simulink model "Target_Control_System"  (R2021b)
settings: Solver=FixedStepDiscrete  StartTime=0.0  StopTime=5  RelTol=1e-3
PreLoadFcn:
  | RTWConfigurationCB('preloadfcn', bdroot);
PostLoadFcn:
  | load('configuration/data_struct.mat');
  | load('configuration/fluxMaps_propMotor.mat');
  | load('configuration/parameterInit_PROP.mat');
  | load('configuration/parameterInit_PUMP.mat');
  | load('configuration/parameterInit_PITCH.mat');
  | load('configuration/parameterInit_TILT.mat');
  | %load('configuration/base_workspace_signal_definition.mat');
  | %load('resolvedatastores_to_baseworkspace_for_faster_simulation.mat');
model workspace (MAT data in the model file):
  SIMULATION_OPTIONS : Simulink.Parameter (value not decoded)
  TARGET_CODE_GEN : Simulink.Parameter (value not decoded)
  TCS_SAMPLE_FREQ_HZ : Simulink.Parameter (value not decoded)
symbols that are objects in the model workspace (value not decoded): TARGET_CODE_GEN, TCS_SAMPLE_FREQ_HZ
undefined symbols (not defined in the file): A_DQ_REF_LPF_INIT__PITCH, A_DQ_REF_LPF_INIT__PROP, A_DQ_REF_LPF_INIT__PUMP, A_DQ_REF_LPF_INIT__TILT, A_OBSERVER_CONFIDENCE_INIT__PITCH, A_OBSERVER_CONFIDENCE_INIT__PROP, A_OBSERVER_CONFIDENCE_INIT__PUMP, A_OBSERVER_CONFIDENCE_INIT__TILT, ACTUATOR_MAX_ANGLE_TRIP__PITCH, ACTUATOR_MIN_ANGLE_TRIP__PITCH, ACTUATOR_POS_SENSOR_INV_DIRECTION__PITCH, ACTUATOR_POS_SENSOR_INV_DIRECTION__TILT, ACTUATOR_POS_SENSOR_OFFSET__PITCH, ACTUATOR_POS_SENSOR_OFFSET__TILT, ADC_scaler1_baseaddr_TILT, ADC_SCALER_FLOAT_TO_FIXPOINT_EXPANSION, ANGLE_ELEC_FROM_SENSOR_OFFSET_INIT__PITCH, ANGLE_ELEC_FROM_SENSOR_OFFSET_INIT__PROP, ANGLE_ELEC_FROM_SENSOR_OFFSET_INIT__PUMP, ANGLE_ELEC_FROM_SENSOR_OFFSET_INIT__TILT, AUTO_CLEAR_FAULTS_ENABLED__PITCH, AUTO_CLEAR_FAULTS_ENABLED__PROP, AUTO_CLEAR_FAULTS_ENABLED__PUMP, AUTO_CLEAR_FAULTS_ENABLED__TILT, AUTO_CLEAR_FAULTS_WAIT_TICKS__PITCH, AUTO_CLEAR_FAULTS_WAIT_TICKS__PROP, AUTO_CLEAR_FAULTS_WAIT_TICKS__PUMP, AUTO_CLEAR_FAULTS_WAIT_TICKS__TILT, AUTO_I_ZERO_IDLE_TICKS__PITCH, AUTO_I_ZERO_IDLE_TICKS__PROP, AUTO_I_ZERO_IDLE_TICKS__PUMP, AUTO_I_ZERO_IDLE_TICKS__TILT, AUTO_I_ZERO_OFFSET_IDC_THRESHOLD__PITCH, AUTO_I_ZERO_OFFSET_IDC_THRESHOLD__PROP, AUTO_I_ZERO_OFFSET_IDC_THRESHOLD__PUMP, AUTO_I_ZERO_OFFSET_IDC_THRESHOLD__TILT, AUTO_I_ZERO_OFFSET_IPH_THRESHOLD__PITCH, AUTO_I_ZERO_OFFSET_IPH_THRESHOLD__PROP, AUTO_I_ZERO_OFFSET_IPH_THRESHOLD__PUMP, AUTO_I_ZERO_OFFSET_IPH_THRESHOLD__TILT, AUTO_SENSORLESS_SWITCHOVER_DISABLE_OMEGA, AUTO_SENSORLESS_SWITCHOVER_ENABLE_OMEGA, AUTO_SENSORLESS_SWITCHOVER_MIN_CONFIDENCE, AUXILIARY_PROTECTION_UNIT_BASEADDR__TILT, blanking_max_error_omega_INIT_PITCH, blanking_max_error_omega_INIT_TILT, blanking_max_error_position_INIT_PITCH, blanking_max_error_position_INIT_TILT, BRUTE_START_I_Q_REF_RAMP_SPEED__PITCH, BRUTE_START_I_Q_REF_RAMP_SPEED__PROP, BRUTE_START_I_Q_REF_RAMP_SPEED__PUMP, BRUTE_START_I_Q_REF_RAMP_SPEED__TILT, CONTROL_LOOP_DT_INIT__PITCH, CONTROL_LOOP_DT_INIT__PROP, CONTROL_LOOP_DT_INIT__PUMP, CONTROL_LOOP_DT_INIT__TILT, CORRECTION_FILTER_SCALE__PITCH, CORRECTION_FILTER_SCALE__PROP, CORRECTION_FILTER_SCALE__PUMP, CORRECTION_FILTER_SCALE__TILT ... (+458)
libraries: simulink x178, Reusables_Lib x24
(part 9 of 47)

== system Target_Control_System/Target_Control_System/Simulation Controls/Simulation Data Store Initialization/setupIirFilters(&oTilt) ==
  setupIirFilters : TriggerPort  TriggerType=function-call  VariantControl=(inherit)  OutputDataType=int8
  Constant : Constant  Value=5000  OutDataTypeStr=single  SampleTime=-1
  Data Store Read : DataStoreRead  DataStoreName=oTilt  DataStoreElements=oTilt.oHw_.fIirDcFInit_  IndexOptions=Index vector (dialog)  Indices=1  OutputSizes=1
  Data Store Read1 : DataStoreRead  DataStoreName=oTilt  DataStoreElements=oTilt.oHw_.fIirFSample_  IndexOptions=Index vector (dialog)  Indices=1  OutputSizes=1
  Data Store Read2 : DataStoreRead  DataStoreName=oTilt  DataStoreElements=oTilt.oHw_.fIirUphaseFInit_  IndexOptions=Index vector (dialog)  Indices=1  OutputSizes=1
  Data Store Read3 : DataStoreRead  DataStoreName=oTilt  DataStoreElements=oTilt.oHw_.fIirIphaseFInit_  IndexOptions=Index vector (dialog)  Indices=1  OutputSizes=1
  Data Store Read5 : DataStoreRead  DataStoreName=oTilt  DataStoreElements=oTilt.oMot_.oState_.fMotorAccelerationStage2Bandwidth_  IndexOptions=Index vector (dialog)  Indices=1  OutputSizes=1
  Data Store Write1 : DataStoreWrite  DataStoreName=oTilt  DataStoreElements=oTilt.oMot_.oParam_.fIdcIirFLpfRads_  IndexOptions=Index vector (dialog)  Indices=1  OutputSizes=1
  Data Store Write11 : DataStoreWrite  DataStoreName=oTilt  DataStoreElements=oTilt.oMot_.oParam_.fUdcIirFLpfRads_  IndexOptions=Index vector (dialog)  Indices=1  OutputSizes=1
  Data Store Write2 : DataStoreWrite  DataStoreName=oTilt  DataStoreElements=oTilt.oMot_.oParam_.fUphaseIirFLpfRads_  IndexOptions=Index vector (dialog)  Indices=1  OutputSizes=1
  Data Store Write3 : DataStoreWrite  DataStoreName=oTilt  DataStoreElements=oTilt.oMot_.oParam_.fIphaseIirFLpfRads_  IndexOptions=Index vector (dialog)  Indices=1  OutputSizes=1
  Data Store Write4 : DataStoreWrite  DataStoreName=oTilt  DataStoreElements=oTilt.oMot_.oState_.fMotorAccelerationStage2Bandwidth_  IndexOptions=Index vector (dialog)  Indices=1  OutputSizes=1
  Gain : Gain  Gain=2*pi
  Gain1 : Gain  Gain=2*pi
  Gain2 : Gain  Gain=2*pi
  computeCoefficientsButter() : Subsystem
  computeCoefficientsButter()1 : Subsystem
  computeCoefficientsButter()2 : Subsystem
  softwareIirFilterInitialize() : Subsystem  Priority=15  TreatAsAtomicUnit=on
  wires:
  Data Store Read/1 -> computeCoefficientsButter()/1(fCutoffFrequencyHz)
  Data Store Read5/1 -> softwareIirFilterInitialize()/1(fFreq3db)
  Gain2/1 -> Data Store Write3/1
  computeCoefficientsButter()2/2(fCutoffFrequencyHz_out) -> Gain2/1
  Data Store Read3/1 -> computeCoefficientsButter()2/1(fCutoffFrequencyHz)
  softwareIirFilterInitialize()/1(fActualFrequencyHz) -> Data Store Write4/1
  computeCoefficientsButter()/2(fCutoffFrequencyHz_out) -> Gain/1
  Data Store Read1/1 -> computeCoefficientsButter()/2(dSampleFrequencyHz), computeCoefficientsButter()1/2(dSampleFrequencyHz), computeCoefficientsButter()2/2(dSampleFrequencyHz)
  Gain1/1 -> Data Store Write2/1
  Gain/1 -> Data Store Write11/1, Data Store Write1/1
  Constant/1 -> softwareIirFilterInitialize()/2(fFreqSample)
  Data Store Read2/1 -> computeCoefficientsButter()1/1(fCutoffFrequencyHz)
  computeCoefficientsButter()1/2(fCutoffFrequencyHz_out) -> Gain1/1

== system Target_Control_System/Target_Control_System/Simulation Controls/Simulation Data Store Initialization/setupIirFilters() ==
  setupIirFilters : TriggerPort  TriggerType=function-call  VariantControl=(inherit)  OutputDataType=int8
  Constant : Constant  Value=5000  OutDataTypeStr=single  SampleTime=-1
  Data Store Read : DataStoreRead  DataStoreName=oPitch  DataStoreElements=oPitch.oHw_.fIirDcFInit_  IndexOptions=Index vector (dialog)  Indices=1  OutputSizes=1
  Data Store Read1 : DataStoreRead  DataStoreName=oPitch  DataStoreElements=oPitch.oHw_.fIirFSample_  IndexOptions=Index vector (dialog)  Indices=1  OutputSizes=1
  Data Store Read2 : DataStoreRead  DataStoreName=oPitch  DataStoreElements=oPitch.oHw_.fIirUphaseFInit_  IndexOptions=Index vector (dialog)  Indices=1  OutputSizes=1
  Data Store Read3 : DataStoreRead  DataStoreName=oPitch  DataStoreElements=oPitch.oHw_.fIirIphaseFInit_  IndexOptions=Index vector (dialog)  Indices=1  OutputSizes=1
  Data Store Read5 : DataStoreRead  DataStoreName=oPitch  DataStoreElements=oPitch.oMot_.oState_.fMotorAccelerationStage2Bandwidth_  IndexOptions=Index vector (dialog)  Indices=1  OutputSizes=1
  Data Store Write1 : DataStoreWrite  DataStoreName=oPitch  DataStoreElements=oPitch.oMot_.oParam_.fIdcIirFLpfRads_  IndexOptions=Index vector (dialog)  Indices=1  OutputSizes=1
  Data Store Write11 : DataStoreWrite  DataStoreName=oPitch  DataStoreElements=oPitch.oMot_.oParam_.fUdcIirFLpfRads_  IndexOptions=Index vector (dialog)  Indices=1  OutputSizes=1
  Data Store Write2 : DataStoreWrite  DataStoreName=oPitch  DataStoreElements=oPitch.oMot_.oParam_.fUphaseIirFLpfRads_  IndexOptions=Index vector (dialog)  Indices=1  OutputSizes=1
  Data Store Write3 : DataStoreWrite  DataStoreName=oPitch  DataStoreElements=oPitch.oMot_.oParam_.fIphaseIirFLpfRads_  IndexOptions=Index vector (dialog)  Indices=1  OutputSizes=1
  Data Store Write4 : DataStoreWrite  DataStoreName=oPitch  DataStoreElements=oPitch.oMot_.oState_.fMotorAccelerationStage2Bandwidth_  IndexOptions=Index vector (dialog)  Indices=1  OutputSizes=1
  Gain : Gain  Gain=2*pi
  Gain1 : Gain  Gain=2*pi
  Gain2 : Gain  Gain=2*pi
  computeCoefficientsButter() : Subsystem
  computeCoefficientsButter()1 : Subsystem
  computeCoefficientsButter()2 : Subsystem
  softwareIirFilterInitialize() : Subsystem  Priority=15  TreatAsAtomicUnit=on
  wires:
  Data Store Read/1 -> computeCoefficientsButter()/1(fCutoffFrequencyHz)
  Data Store Read5/1 -> softwareIirFilterInitialize()/1(fFreq3db)
  Gain2/1 -> Data Store Write3/1
  computeCoefficientsButter()2/2(fCutoffFrequencyHz_out) -> Gain2/1
  Data Store Read3/1 -> computeCoefficientsButter()2/1(fCutoffFrequencyHz)
  softwareIirFilterInitialize()/1(fActualFrequencyHz) -> Data Store Write4/1
  computeCoefficientsButter()/2(fCutoffFrequencyHz_out) -> Gain/1
  Data Store Read1/1 -> computeCoefficientsButter()/2(dSampleFrequencyHz), computeCoefficientsButter()1/2(dSampleFrequencyHz), computeCoefficientsButter()2/2(dSampleFrequencyHz)
  Gain1/1 -> Data Store Write2/1
  Gain/1 -> Data Store Write11/1, Data Store Write1/1
  Constant/1 -> softwareIirFilterInitialize()/2(fFreqSample)
  Data Store Read2/1 -> computeCoefficientsButter()1/1(fCutoffFrequencyHz)
  computeCoefficientsButter()1/2(fCutoffFrequencyHz_out) -> Gain1/1

== system Target_Control_System/Target_Control_System/Simulation Controls/Simulation Data Store Initialization/setupObserver(&oTilt) ==
  setupObserver_Tilt : TriggerPort  TriggerType=function-call  VariantControl=Variant
  Data Store Read : DataStoreRead  DataStoreName=oTilt  DataStoreElements=oTilt.oIsr_.oParam_  IndexOptions=Index vector (dialog)  Indices=1  OutputSizes=1
  Data Store Read1 : DataStoreRead  DataStoreName=oTilt  DataStoreElements=oTilt.oMot_.oParam_  IndexOptions=Index vector (dialog)  Indices=1  OutputSizes=1
  Data Store Write : DataStoreWrite  DataStoreName=oTilt  DataStoreElements=oTilt.oIsr_.oParam_  IndexOptions=Index vector (dialog)  Indices=1  OutputSizes=1
  Data Store Write1 : DataStoreWrite  DataStoreName=oTilt  DataStoreElements=oTilt.oMot_.oParam_  IndexOptions=Index vector (dialog)  Indices=1  OutputSizes=1
  updateObserver_port() : Reusables_Lib/updateObserver_port()  Priority=10  SystemSampleTime=-1  VariantActivationTime=update diagram  Latency=0  AutoFrameSizeCalculation=off
  wires:
  Data Store Read/1 -> updateObserver_port()/1
  Data Store Read1/1 -> updateObserver_port()/2
  updateObserver_port()/1 -> Data Store Write/1
  updateObserver_port()/2 -> Data Store Write1/1

== system Target_Control_System/Target_Control_System/Simulation Controls/Simulation Data Store Initialization/setupObserver() ==
  setupObserver : TriggerPort  TriggerType=function-call  VariantControl=(inherit)  OutputDataType=int8
  Constant : Constant  Value=50000  OutDataTypeStr=single  SampleTime=-1
  Data Store Read : DataStoreRead  DataStoreName=oPitch  DataStoreElements=oPitch.oIsr_.oParam_.fObserverMaxOmegaE_  IndexOptions=Index vector (dialog)  Indices=1  OutputSizes=1
  Data Store Read1 : DataStoreRead  DataStoreName=oPitch  DataStoreElements=oPitch.oIsr_.oParam_.fObserverMaxOmegaEAccel_  IndexOptions=Index vector (dialog)  Indices=1  OutputSizes=1
  Data Store Read2 : DataStoreRead  Priority=5  DataStoreName=oPitch  DataStoreElements=oPitch.oIsr_.oParam_.fControlLoopDt_  IndexOptions=Index vector (dialog)  Indices=1  OutputSizes=1
  Data Store Read3 : DataStoreRead  Priority=5  DataStoreName=oPitch  DataStoreElements=oPitch.oMot_.oParam_.fObserverLoopFilterBandwidthHz_  IndexOptions=Index vector (dialog)  Indices=1  OutputSizes=1
  Data Store Write : DataStoreWrite  DataStoreName=oPitch  DataStoreElements=oPitch.oIsr_.oParam_.oPiDataPll2_.oParameter_.fIntMax_  IndexOptions=Index vector (dialog)  Indices=1  OutputSizes=1
  Data Store Write1 : DataStoreWrite  DataStoreName=oPitch  DataStoreElements=oPitch.oIsr_.oParam_.oPiDataPll2_.oParameter_.fIntMin_  IndexOptions=Index vector (dialog)  Indices=1  OutputSizes=1
  Data Store Write2 : DataStoreWrite  DataStoreName=oPitch  DataStoreElements=oPitch.oIsr_.oParam_.oPiDataPll2_.oParameter_.fOutMin_  IndexOptions=Index vector (dialog)  Indices=1  OutputSizes=1
  Data Store Write3 : DataStoreWrite  DataStoreName=oPitch  DataStoreElements=oPitch.oIsr_.oParam_.oPiDataPll2_.oParameter_.fOutMax_  IndexOptions=Index vector (dialog)  Indices=1  OutputSizes=1
  Data Store Write4 : DataStoreWrite  DataStoreName=oPitch  DataStoreElements=oPitch.oIsr_.oParam_.oPiDataPll2_.oParameter_.fKi_  IndexOptions=Index vector (dialog)  Indices=1  OutputSizes=1
  Gain : Gain  Gain=-1
  Gain1 : Gain  Gain=-1
  updateObserver()_pitch : Subsystem  Priority=10  TreatAsAtomicUnit=on
  wires:
  Gain/1 -> Data Store Write1/1
  Gain1/1 -> Data Store Write2/1
  Data Store Read2/1 -> updateObserver()_pitch/1(oIsr_.oParam_.fControlLoopDt_)
  Data Store Read1/1 -> Gain1/1, Data Store Write3/1
  Constant/1 -> Data Store Write4/1
  Data Store Read/1 -> Gain/1, Data Store Write/1
  Data Store Read3/1 -> updateObserver()_pitch/2(fObserverLoopFilterBandwidthHz_)

== system Target_Control_System/Target_Control_System/Simulation Controls/Simulation Data Store Initialization/setupObserverForPosSensor(&oTilt) ==
  setupObserverForPosSensor : TriggerPort  TriggerType=function-call  VariantControl=(inherit)  OutputDataType=int8
  Data Store Read : DataStoreRead  DataStoreName=oTilt  DataStoreElements=oTilt.oMot_.oParam_.fIntControlLoopDt_  IndexOptions=Index vector (dialog)  Indices=1  OutputSizes=1
  Data Store Read1 : DataStoreRead  DataStoreName=oTilt  DataStoreElements=oTilt.oMot_.oState_.oPosSensor_.fOmegaEDifferentiatorBandwidthHz_  IndexOptions=Index vector (dialog)  Indices=1  OutputSizes=1
  Data Store Write : DataStoreWrite  DataStoreName=oTilt  DataStoreElements=oTilt.oMot_.oState_.oPosSensor_.fOmegaEDifferentiatorBandwidthHz_  IndexOptions=Index vector (dialog)  Indices=1  OutputSizes=1
  softwareIirFilterInitialize() : Subsystem  TreatAsAtomicUnit=on
  wires:
  Data Store Read1/1 -> softwareIirFilterInitialize()/1(fFreq3db)
  softwareIirFilterInitialize()/1(fActualFrequencyHz) -> Data Store Write/1
  Data Store Read/1 -> softwareIirFilterInitialize()/2(fControlLoopDt_)

== system Target_Control_System/Target_Control_System/Simulation Controls/Simulation Data Store Initialization/setupPwm(&oTilt) ==
  setupPwm : TriggerPort  TriggerType=function-call  VariantControl=(inherit)  OutputDataType=int8
  Constant : Constant  Priority=-1  OutDataTypeStr=uint32  SampleTime=-1
  Constant1 : Constant  Priority=-1  Value=0  OutDataTypeStr=uint32  SampleTime=-1
  Data Store Read : DataStoreRead  Priority=-1  DataStoreName=oTilt  DataStoreElements=oTilt.oMot_.oParam_.fPwmFreqKhz_  IndexOptions=Index vector (dialog)  Indices=1  OutputSizes=1
  Data Store Read1 : DataStoreRead  Priority=-1  DataStoreName=oTilt  DataStoreElements=oTilt.oMot_.oState_.fMotorAccelerationStage1Bandwidth_  IndexOptions=Index vector (dialog)  Indices=1  OutputSizes=1
  Data Store Read2 : DataStoreRead  Priority=-1  DataStoreName=oTilt  DataStoreElements=oTilt.oMot_.oState_.fFilterBandwidthForSpeedControlIqRef_  IndexOptions=Index vector (dialog)  Indices=1  OutputSizes=1
  Data Store Write : DataStoreWrite  Priority=-1  DataStoreName=oTilt  DataStoreElements=oTilt.oMot_.oOut_.uiPwmRequestFromMain_  IndexOptions=Index vector (dialog)  Indices=1  OutputSizes=1
  Data Store Write1 : DataStoreWrite  Priority=-1  DataStoreName=oTilt  DataStoreElements=oTilt.oMot_.oOut_.uiPwmDutyTicksFromMainA_  IndexOptions=Index vector (dialog)  Indices=1  OutputSizes=1
  Data Store Write2 : DataStoreWrite  Priority=-1  DataStoreName=oTilt  DataStoreElements=oTilt.oMot_.oOut_.uiPwmDutyTicksFromMainB_  IndexOptions=Index vector (dialog)  Indices=1  OutputSizes=1
  Data Store Write4 : DataStoreWrite  Priority=-1  DataStoreName=oTilt  DataStoreElements=oTilt.oMot_.oOut_.uiPwmDutyTicksFromMainC_  IndexOptions=Index vector (dialog)  Indices=1  OutputSizes=1
  setPwmFrequencyApplication()_tilt : Subsystem  Priority=1  TreatAsAtomicUnit=on
  wires:
  Data Store Read/1 -> setPwmFrequencyApplication()_tilt/1(fPwmFreqKhz_)
  Data Store Read1/1 -> setPwmFrequencyApplication()_tilt/2(fMotorAccelerationStage1Bandwidth_)
  Data Store Read2/1 -> setPwmFrequencyApplication()_tilt/3(fFilterBandwidthForSpeedControlIqRef_)
  Constant1/1 -> Data Store Write1/1, Data Store Write2/1, Data Store Write4/1
  Constant/1 -> Data Store Write/1

== system Target_Control_System/Target_Control_System/Simulation Controls/Simulation Data Store Initialization/setupPwm() ==
  setupPwm : TriggerPort  TriggerType=function-call  VariantControl=(inherit)  OutputDataType=int8
  Constant : Constant  Priority=-1  OutDataTypeStr=uint32  SampleTime=-1
  Constant1 : Constant  Priority=-1  Value=0  OutDataTypeStr=uint32  SampleTime=-1
  Data Store Read : DataStoreRead  Priority=-1  DataStoreName=oPitch  DataStoreElements=oPitch.oMot_.oParam_.fPwmFreqKhz_  IndexOptions=Index vector (dialog)  Indices=1  OutputSizes=1
  Data Store Read1 : DataStoreRead  Priority=-1  DataStoreName=oPitch  DataStoreElements=oPitch.oMot_.oState_.fMotorAccelerationStage1Bandwidth_  IndexOptions=Index vector (dialog)  Indices=1  OutputSizes=1
  Data Store Read2 : DataStoreRead  Priority=-1  DataStoreName=oPitch  DataStoreElements=oPitch.oMot_.oState_.fFilterBandwidthForSpeedControlIqRef_  IndexOptions=Index vector (dialog)  Indices=1  OutputSizes=1
  Data Store Write : DataStoreWrite  Priority=-1  DataStoreName=oPitch  DataStoreElements=oPitch.oMot_.oOut_.uiPwmRequestFromMain_  IndexOptions=Index vector (dialog)  Indices=1  OutputSizes=1
  Data Store Write1 : DataStoreWrite  Priority=-1  DataStoreName=oPitch  DataStoreElements=oPitch.oMot_.oOut_.uiPwmDutyTicksFromMainA_  IndexOptions=Index vector (dialog)  Indices=1  OutputSizes=1
  Data Store Write2 : DataStoreWrite  Priority=-1  DataStoreName=oPitch  DataStoreElements=oPitch.oMot_.oOut_.uiPwmDutyTicksFromMainB_  IndexOptions=Index vector (dialog)  Indices=1  OutputSizes=1
  Data Store Write4 : DataStoreWrite  Priority=-1  DataStoreName=oPitch  DataStoreElements=oPitch.oMot_.oOut_.uiPwmDutyTicksFromMainC_  IndexOptions=Index vector (dialog)  Indices=1  OutputSizes=1
  setPwmFrequencyApplication()_pitch : Subsystem  Priority=1  TreatAsAtomicUnit=on
  wires:
  Data Store Read/1 -> setPwmFrequencyApplication()_pitch/1(fPwmFreqKhz_)
  Data Store Read1/1 -> setPwmFrequencyApplication()_pitch/2(fMotorAccelerationStage1Bandwidth_)
  Data Store Read2/1 -> setPwmFrequencyApplication()_pitch/3(fFilterBandwidthForSpeedControlIqRef_)
  Constant1/1 -> Data Store Write1/1, Data Store Write2/1, Data Store Write4/1
  Constant/1 -> Data Store Write/1

== system Target_Control_System/Target_Control_System/Simulation Controls/Simulation Data Store Initialization/updateIqSetpointMax(&oTilt) ==
  updateIqSetpointMax : TriggerPort  TriggerType=function-call  VariantControl=(inherit)  OutputDataType=int8
  Add : Sum
  Constant : Constant  OutDataTypeStr=single  SampleTime=-1
  Constant1 : Constant  Value=0  OutDataTypeStr=single  SampleTime=-1
  Constant2 : Constant  Value=0  OutDataTypeStr=single  SampleTime=-1
  Data Store Read : DataStoreRead  DataStoreName=oTilt  DataStoreElements=oTilt.oMot_.oParam_.fISetpointMax_  IndexOptions=Index vector (dialog)  Indices=1  OutputSizes=1
  Data Store Read1 : DataStoreRead  DataStoreName=oTilt  DataStoreElements=oTilt.oMot_.oParam_.fIdRefFractionOfIq_  IndexOptions=Index vector (dialog)  Indices=1  OutputSizes=1
  Data Store Read2 : DataStoreRead  DataStoreName=oTilt  DataStoreElements=oTilt.oMot_.oParam_.fTorqueAuthorityFraction_  IndexOptions=Index vector (dialog)  Indices=1  OutputSizes=1
  Data Store Read3 : DataStoreRead  DataStoreName=oTilt  DataStoreElements=oTilt.oMot_.oParam_.oPiDataRpm_.oParameter_.fIntMin_  IndexOptions=Index vector (dialog)  Indices=1  OutputSizes=1
  Data Store Read4 : DataStoreRead  DataStoreName=oTilt  DataStoreElements=oTilt.oMot_.oParam_.oPiDataRpm_.oParameter_.fOutMin_  IndexOptions=Index vector (dialog)  Indices=1  OutputSizes=1
  Data Store Write : DataStoreWrite  DataStoreName=oTilt  DataStoreElements=oTilt.oMot_.oParam_.fIqSetpointMax_  IndexOptions=Index vector (dialog)  Indices=1  OutputSizes=1
  Data Store Write1 : DataStoreWrite  DataStoreName=oTilt  DataStoreElements=oTilt.oMot_.oParam_.oPiDataRpm_.oParameter_.fIntMax_  IndexOptions=Index vector (dialog)  Indices=1  OutputSizes=1
  Data Store Write10 : DataStoreWrite  DataStoreName=oTilt  DataStoreElements=oTilt.oMot_.oParam_.oPid2DataRpmCtrl_.oParameter_.fDMax_  IndexOptions=Index vector (dialog)  Indices=1  OutputSizes=1
  Data Store Write2 : DataStoreWrite  DataStoreName=oTilt  DataStoreElements=oTilt.oMot_.oParam_.oPiDataRpm_.oParameter_.fIntMin_  IndexOptions=Index vector (dialog)  Indices=1  OutputSizes=1
  Data Store Write3 : DataStoreWrite  DataStoreName=oTilt  DataStoreElements=oTilt.oMot_.oParam_.oPiDataRpm_.oParameter_.fOutMax_  IndexOptions=Index vector (dialog)  Indices=1  OutputSizes=1
  Data Store Write4 : DataStoreWrite  DataStoreName=oTilt  DataStoreElements=oTilt.oMot_.oParam_.oPiDataRpm_.oParameter_.fOutMin_  IndexOptions=Index vector (dialog)  Indices=1  OutputSizes=1
  Data Store Write5 : DataStoreWrite  DataStoreName=oTilt  DataStoreElements=oTilt.oMot_.oParam_.oPid2DataRpmCtrl_.oParameter_.fIntMin_  IndexOptions=Index vector (dialog)  Indices=1  OutputSizes=1
  Data Store Write6 : DataStoreWrite  DataStoreName=oTilt  DataStoreElements=oTilt.oMot_.oParam_.oPid2DataRpmCtrl_.oParameter_.fIntMax_  IndexOptions=Index vector (dialog)  Indices=1  OutputSizes=1
  Data Store Write7 : DataStoreWrite  DataStoreName=oTilt  DataStoreElements=oTilt.oMot_.oParam_.oPid2DataRpmCtrl_.oParameter_.fOutMin_  IndexOptions=Index vector (dialog)  Indices=1  OutputSizes=1
  Data Store Write8 : DataStoreWrite  DataStoreName=oTilt  DataStoreElements=oTilt.oMot_.oParam_.oPid2DataRpmCtrl_.oParameter_.fOutMax_  IndexOptions=Index vector (dialog)  Indices=1  OutputSizes=1
  Data Store Write9 : DataStoreWrite  DataStoreName=oTilt  DataStoreElements=oTilt.oMot_.oParam_.oPid2DataRpmCtrl_.oParameter_.fDMin_  IndexOptions=Index vector (dialog)  Indices=1  OutputSizes=1
  Divide : Product  Inputs=**
  Divide1 : Product  Inputs=**/
  Gain{,1..4} (5 alike) : Gain  Gain=-1
  Relational Operator : RelationalOperator  Operator===  OutDataTypeStr=boolean  RndMeth=Simplest
  Relational Operator1 : RelationalOperator  Operator===  OutDataTypeStr=boolean  RndMeth=Simplest
  Sqrt : Sqrt  SaturateOnIntegerOverflow=on
  Switch : Switch  Criteria=u2 > Threshold
  Switch1 : Switch  Criteria=u2 > Threshold
  wires:
  Sqrt/1 -> Divide1/3
  Data Store Read3/1 -> Relational Operator/1, Switch/1
  Data Store Read1/1 -> Divide/1, Divide/2
  Data Store Read/1 -> Divide1/2
  Constant1/1 -> Relational Operator/2
  Add/1 -> Sqrt/1
  Constant/1 -> Add/2
  Relational Operator1/1 -> Switch1/2
  Gain/1 -> Switch/3
  Divide1/1 -> Data Store Write3/1, Data Store Write6/1, Data Store Write8/1, Data Store Write10/1, Gain4/1, Gain3/1, Gain2/1, Data Store Write1/1, Data Store Write/1, Gain/1, Gain1/1
  Relational Operator/1 -> Switch/2
  Divide/1 -> Add/1
  Switch1/1 -> Data Store Write4/1
  Switch/1 -> Data Store Write2/1
  Constant2/1 -> Relational Operator1/2
  Data Store Read4/1 -> Relational Operator1/1, Switch1/1
  Gain4/1 -> Data Store Write9/1
  Gain1/1 -> Switch1/3
  Gain3/1 -> Data Store Write7/1
  Data Store Read2/1 -> Divide1/1
  Gain2/1 -> Data Store Write5/1

== system Target_Control_System/Target_Control_System/Simulation Controls/Simulation Data Store Initialization/updateIqSetpointMax() ==
  updateIqSetpointMax : TriggerPort  TriggerType=function-call  VariantControl=(inherit)  OutputDataType=int8
  Add : Sum
  Constant : Constant  OutDataTypeStr=single  SampleTime=-1
  Constant1 : Constant  Value=0  OutDataTypeStr=single  SampleTime=-1
  Constant2 : Constant  Value=0  OutDataTypeStr=single  SampleTime=-1
  Data Store Read : DataStoreRead  DataStoreName=oPitch  DataStoreElements=oPitch.oMot_.oParam_.fISetpointMax_  IndexOptions=Index vector (dialog)  Indices=1  OutputSizes=1
  Data Store Read1 : DataStoreRead  DataStoreName=oPitch  DataStoreElements=oPitch.oMot_.oParam_.fIdRefFractionOfIq_  IndexOptions=Index vector (dialog)  Indices=1  OutputSizes=1
  Data Store Read2 : DataStoreRead  DataStoreName=oPitch  DataStoreElements=oPitch.oMot_.oParam_.fTorqueAuthorityFraction_  IndexOptions=Index vector (dialog)  Indices=1  OutputSizes=1
  Data Store Read3 : DataStoreRead  DataStoreName=oPitch  DataStoreElements=oPitch.oMot_.oParam_.oPiDataRpm_.oParameter_.fIntMin_  IndexOptions=Index vector (dialog)  Indices=1  OutputSizes=1
  Data Store Read4 : DataStoreRead  DataStoreName=oPitch  DataStoreElements=oPitch.oMot_.oParam_.oPiDataRpm_.oParameter_.fOutMin_  IndexOptions=Index vector (dialog)  Indices=1  OutputSizes=1
  Data Store Write : DataStoreWrite  DataStoreName=oPitch  DataStoreElements=oPitch.oMot_.oParam_.fIqSetpointMax_  IndexOptions=Index vector (dialog)  Indices=1  OutputSizes=1
  Data Store Write1 : DataStoreWrite  DataStoreName=oPitch  DataStoreElements=oPitch.oMot_.oParam_.oPiDataRpm_.oParameter_.fIntMax_  IndexOptions=Index vector (dialog)  Indices=1  OutputSizes=1
  Data Store Write10 : DataStoreWrite  DataStoreName=oPitch  DataStoreElements=oPitch.oMot_.oParam_.oPid2DataRpmCtrl_.oParameter_.fDMax_  IndexOptions=Index vector (dialog)  Indices=1  OutputSizes=1
  Data Store Write2 : DataStoreWrite  DataStoreName=oPitch  DataStoreElements=oPitch.oMot_.oParam_.oPiDataRpm_.oParameter_.fIntMin_  IndexOptions=Index vector (dialog)  Indices=1  OutputSizes=1
  Data Store Write3 : DataStoreWrite  DataStoreName=oPitch  DataStoreElements=oPitch.oMot_.oParam_.oPiDataRpm_.oParameter_.fOutMax_  IndexOptions=Index vector (dialog)  Indices=1  OutputSizes=1
  Data Store Write4 : DataStoreWrite  DataStoreName=oPitch  DataStoreElements=oPitch.oMot_.oParam_.oPiDataRpm_.oParameter_.fOutMin_  IndexOptions=Index vector (dialog)  Indices=1  OutputSizes=1
  Data Store Write5 : DataStoreWrite  DataStoreName=oPitch  DataStoreElements=oPitch.oMot_.oParam_.oPid2DataRpmCtrl_.oParameter_.fIntMin_  IndexOptions=Index vector (dialog)  Indices=1  OutputSizes=1
  Data Store Write6 : DataStoreWrite  DataStoreName=oPitch  DataStoreElements=oPitch.oMot_.oParam_.oPid2DataRpmCtrl_.oParameter_.fIntMax_  IndexOptions=Index vector (dialog)  Indices=1  OutputSizes=1
  Data Store Write7 : DataStoreWrite  DataStoreName=oPitch  DataStoreElements=oPitch.oMot_.oParam_.oPid2DataRpmCtrl_.oParameter_.fOutMin_  IndexOptions=Index vector (dialog)  Indices=1  OutputSizes=1
  Data Store Write8 : DataStoreWrite  DataStoreName=oPitch  DataStoreElements=oPitch.oMot_.oParam_.oPid2DataRpmCtrl_.oParameter_.fOutMax_  IndexOptions=Index vector (dialog)  Indices=1  OutputSizes=1
  Data Store Write9 : DataStoreWrite  DataStoreName=oPitch  DataStoreElements=oPitch.oMot_.oParam_.oPid2DataRpmCtrl_.oParameter_.fDMin_  IndexOptions=Index vector (dialog)  Indices=1  OutputSizes=1
  Divide : Product  Inputs=**
  Divide1 : Product  Inputs=**/
  Gain{,1..4} (5 alike) : Gain  Gain=-1
  Relational Operator : RelationalOperator  Operator===  OutDataTypeStr=boolean  RndMeth=Simplest
  Relational Operator1 : RelationalOperator  Operator===  OutDataTypeStr=boolean  RndMeth=Simplest
  Sqrt : Sqrt  SaturateOnIntegerOverflow=on
  Switch : Switch  Criteria=u2 > Threshold
  Switch1 : Switch  Criteria=u2 > Threshold
  wires:
  Sqrt/1 -> Divide1/3
  Data Store Read3/1 -> Relational Operator/1, Switch/1
  Data Store Read1/1 -> Divide/1, Divide/2
  Data Store Read/1 -> Divide1/2
  Constant1/1 -> Relational Operator/2
  Add/1 -> Sqrt/1
  Constant/1 -> Add/2
  Relational Operator1/1 -> Switch1/2
  Gain/1 -> Switch/3
  Divide1/1 -> Data Store Write3/1, Data Store Write6/1, Data Store Write8/1, Data Store Write10/1, Gain4/1, Gain3/1, Gain2/1, Data Store Write1/1, Data Store Write/1, Gain/1, Gain1/1
  Relational Operator/1 -> Switch/2
  Divide/1 -> Add/1
  Switch1/1 -> Data Store Write4/1
  Switch/1 -> Data Store Write2/1
  Constant2/1 -> Relational Operator1/2
  Data Store Read4/1 -> Relational Operator1/1, Switch1/1
  Gain4/1 -> Data Store Write9/1
  Gain1/1 -> Switch1/3
  Gain3/1 -> Data Store Write7/1
  Data Store Read2/1 -> Divide1/1
  Gain2/1 -> Data Store Write5/1

== system Target_Control_System/Target_Control_System/Simulation Controls/Simulation Data Store Initialization/updateServoObserver(&oTilt) ==
  updateServoObserver : TriggerPort  TriggerType=function-call  VariantControl=(inherit)  OutputDataType=int8
  Data Store Read : DataStoreRead  DataStoreName=oTilt  DataStoreElements=oTilt.oMot_.oParam_.fIntControlLoopDt_  IndexOptions=Index vector (dialog)  Indices=1  OutputSizes=1
  Data Store Read1 : DataStoreRead  DataStoreName=oTilt  DataStoreElements=oTilt.oMot_.oState_.oPosSensor_.fOmegaEDifferentiatorBandwidthHz_  IndexOptions=Index vector (dialog)  Indices=1  OutputSizes=1
  updateServoObserver() : Subsystem  Priority=10  TreatAsAtomicUnit=on
  wires:
  Data Store Read1/1 -> updateServoObserver()/2(fOmegaEDifferentiatorBandwidthHz_)
  Data Store Read/1 -> updateServoObserver()/1(oIsr_.oParam_.fControlLoopDt_)

== system Target_Control_System/Target_Control_System/Simulation Controls/Simulation Data Store Initialization/updateServoObserver() ==
  updateServoObserver : TriggerPort  TriggerType=function-call  VariantControl=(inherit)  OutputDataType=int8
  Data Store Read : DataStoreRead  DataStoreName=oPitch  DataStoreElements=oPitch.oMot_.oParam_.fIntControlLoopDt_  IndexOptions=Index vector (dialog)  Indices=1  OutputSizes=1
  Data Store Read1 : DataStoreRead  DataStoreName=oPitch  DataStoreElements=oPitch.oMot_.oState_.oPosSensor_.fOmegaEDifferentiatorBandwidthHz_  IndexOptions=Index vector (dialog)  Indices=1  OutputSizes=1
  updateServoObserver()_pitch : Subsystem  Priority=10  TreatAsAtomicUnit=on
  wires:
  Data Store Read1/1 -> updateServoObserver()_pitch/2(fOmegaEDifferentiatorBandwidthHz_)
  Data Store Read/1 -> updateServoObserver()_pitch/1(oIsr_.oParam_.fControlLoopDt_)

== system Target_Control_System/Target_Control_System/Simulation Controls/Simulation Data Store Initialization/updateSoftCurrentLimitTilt()1 ==
  updateSoftCurrentLimitTilt : TriggerPort  TriggerType=function-call  VariantControl=Variant

== system Target_Control_System/Target_Control_System/Simulation Controls/pitchMotor/Apply Simulation Parameter Values ==
  OneOverSensorPolePairs : Inport
  Data Store Write : DataStoreWrite  DataStoreName=oPitch  DataStoreElements=oPitch.oMot_.oParam_.fOneOverSensorPolepairs_  IndexOptions=Index vector (dialog)  Indices=1  OutputSizes=1
  wires:
  OneOverSensorPolePairs/1 -> Data Store Write/1

== system Target_Control_System/Target_Control_System/Simulation Controls/pitchMotor/Apply Simulation Setpoints ==
  controllerSelection : Inport
  Current Setpoint for Simulation : Inport  Port=2
  Speed Setpoint for Simulation : Inport  Port=3
  Position Setpoint for Simulation : Inport  Port=4
  Constant : Constant  OutDataTypeStr=uint32  SampleTime=-1
  Constant1 : Constant  Value=3  OutDataTypeStr=uint32  SampleTime=-1
  Constant3 : Constant  Value=2  OutDataTypeStr=uint32  SampleTime=-1
  Equal : RelationalOperator  Operator===  OutDataTypeStr=boolean  RndMeth=Simplest
  Equal1 : RelationalOperator  Operator===  OutDataTypeStr=boolean  RndMeth=Simplest
  Equal2 : RelationalOperator  Operator===  OutDataTypeStr=boolean  RndMeth=Simplest
  Set Current : Subsystem  TreatAsAtomicUnit=on
  Set Position : Subsystem  TreatAsAtomicUnit=on
  Set Speed : Subsystem  TreatAsAtomicUnit=on
  wires:
  Position Setpoint for Simulation/1 -> Set Position/1(Position Setpoint for Simulation)
  Speed Setpoint for Simulation/1 -> Set Speed/1(Speed Setpoint for Simulation)
  Current Setpoint for Simulation/1 -> Set Current/1(Current Setpoint for Simulation)
  Equal2/1 -> Set Position/Enable
  Constant1/1 -> Equal2/2
  controllerSelection/1 -> Equal/1, Equal1/1, Equal2/1
  Equal1/1 -> Set Speed/Enable
  Constant3/1 -> Equal1/2
  Constant/1 -> Equal/2
  Equal/1 -> Set Current/Enable

== system Target_Control_System/Target_Control_System/Simulation Controls/pitchMotor/Drive Enable ==
  pitchMotor_uiEnable : Inport
  Trigger : TriggerPort  TriggerType=falling  VariantControl=Variant
  Data Store Write43 : DataStoreWrite  DataStoreName=oPitch  DataStoreElements=oPitch.oMot_.oOut_.uiEnable_  IndexOptions=Index vector (dialog)  Indices=1  OutputSizes=1
  wires:
  pitchMotor_uiEnable/1 -> Data Store Write43/1

== system Target_Control_System/Target_Control_System/Simulation Controls/pitchMotor/Initialize controller ==
  controllerSelection : Inport
  Trigger : TriggerPort  TriggerType=falling  VariantControl=Variant  PortDimensions=1
  Constant : Constant  OutDataTypeStr=uint32  SampleTime=-1
  Constant1 : Constant  Value=3  OutDataTypeStr=uint32  SampleTime=-1
  Constant3 : Constant  Value=2  OutDataTypeStr=uint32  SampleTime=-1
  Equal : RelationalOperator  Operator===  OutDataTypeStr=boolean  RndMeth=Simplest
  Equal1 : RelationalOperator  Operator===  OutDataTypeStr=boolean  RndMeth=Simplest
  Equal2 : RelationalOperator  Operator===  OutDataTypeStr=boolean  RndMeth=Simplest
  Set Current Controller : Subsystem  TreatAsAtomicUnit=on
  Set Position Controller : Subsystem  TreatAsAtomicUnit=on
  Set Speed Controller : Subsystem  TreatAsAtomicUnit=on
  wires:
  Equal2/1 -> Set Position Controller/Enable
  Constant1/1 -> Equal2/2
  controllerSelection/1 -> Equal/1, Equal1/1, Equal2/1
  Equal1/1 -> Set Speed Controller/Enable
  Constant3/1 -> Equal1/2
  Constant/1 -> Equal/2
  Equal/1 -> Set Current Controller/Enable

== system Target_Control_System/Target_Control_System/Simulation Controls/propMotor/Drive Enable ==
  propMotor_uiEnable : Inport
  Trigger : TriggerPort  TriggerType=falling  VariantControl=Variant
  Data Store Write43 : DataStoreWrite  DataStoreName=oProp  DataStoreElements=oProp.oMot_.oOut_.uiEnable_  IndexOptions=Index vector (dialog)  Indices=1  OutputSizes=1
  wires:
  propMotor_uiEnable/1 -> Data Store Write43/1

== system Target_Control_System/Target_Control_System/Simulation Controls/pumpMotor/Drive Enable ==
  pumpMotor_uiEnable : Inport
  Trigger : TriggerPort  TriggerType=falling  VariantControl=Variant
  Data Store Write43 : DataStoreWrite  DataStoreName=oPump  DataStoreElements=oPump.oMot_.oOut_.uiEnable_  IndexOptions=Index vector (dialog)  Indices=1  OutputSizes=1
  wires:
  pumpMotor_uiEnable/1 -> Data Store Write43/1

== system Target_Control_System/Target_Control_System/Simulation Controls/tiltMotor/Apply Simulation Parameter Values ==
  OneOverSensorPolePairs : Inport
  TiltReadheadCompensationEnabled : Inport  Port=2
  Data Store Write : DataStoreWrite  DataStoreName=oTilt  DataStoreElements=oTilt.oMot_.oParam_.fOneOverSensorPolepairs_  IndexOptions=Index vector (dialog)  Indices=1  OutputSizes=1
  Data Store Write1 : DataStoreWrite  DataStoreName=oTilt  DataStoreElements=oTilt.oMot_.oState_.oPosSensor_.iTiltReadheadCompensationEnabled_  IndexOptions=Index vector (dialog)  Indices=1  OutputSizes=1
  wires:
  TiltReadheadCompensationEnabled/1 -> Data Store Write1/1
  OneOverSensorPolePairs/1 -> Data Store Write/1

== system Target_Control_System/Target_Control_System/Simulation Controls/tiltMotor/Apply Simulation Setpoints ==
  controllerSelection : Inport
  Current Setpoint for Simulation : Inport  Port=2
  Speed Setpoint for Simulation : Inport  Port=3
  Position Setpoint for Simulation : Inport  Port=4
  Constant : Constant  OutDataTypeStr=uint32  SampleTime=-1
  Constant1 : Constant  Value=3  OutDataTypeStr=uint32  SampleTime=-1
  Constant3 : Constant  Value=2  OutDataTypeStr=uint32  SampleTime=-1
  Equal : RelationalOperator  Operator===  OutDataTypeStr=boolean  RndMeth=Simplest
  Equal1 : RelationalOperator  Operator===  OutDataTypeStr=boolean  RndMeth=Simplest
  Equal2 : RelationalOperator  Operator===  OutDataTypeStr=boolean  RndMeth=Simplest
  Set Current : Subsystem  TreatAsAtomicUnit=on
  Set Position : Subsystem  TreatAsAtomicUnit=on
  Set Speed : Subsystem  TreatAsAtomicUnit=on
  wires:
  Position Setpoint for Simulation/1 -> Set Position/1(Position Setpoint for Simulation)
  Speed Setpoint for Simulation/1 -> Set Speed/1(Speed Setpoint for Simulation)
  Current Setpoint for Simulation/1 -> Set Current/1(Current Setpoint for Simulation)
  Equal2/1 -> Set Position/Enable
  Constant1/1 -> Equal2/2
  controllerSelection/1 -> Equal/1, Equal1/1, Equal2/1
  Equal1/1 -> Set Speed/Enable
  Constant3/1 -> Equal1/2
  Constant/1 -> Equal/2
  Equal/1 -> Set Current/Enable

== system Target_Control_System/Target_Control_System/Simulation Controls/tiltMotor/Drive Enable ==
  tiltMotor_uiEnable : Inport
  Trigger : TriggerPort  TriggerType=falling  VariantControl=Variant
  Data Store Write43 : DataStoreWrite  DataStoreName=oTilt  DataStoreElements=oTilt.oMot_.oOut_.uiEnable_  IndexOptions=Index vector (dialog)  Indices=1  OutputSizes=1
  wires:
  tiltMotor_uiEnable/1 -> Data Store Write43/1

== system Target_Control_System/Target_Control_System/Simulation Controls/tiltMotor/Initialize controller ==
  controllerSelection : Inport
  Trigger : TriggerPort  TriggerType=falling  VariantControl=Variant  PortDimensions=1
  Constant : Constant  OutDataTypeStr=uint32  SampleTime=-1
  Constant1 : Constant  Value=3  OutDataTypeStr=uint32  SampleTime=-1
  Constant3 : Constant  Value=2  OutDataTypeStr=uint32  SampleTime=-1
  Equal : RelationalOperator  Operator===  OutDataTypeStr=boolean  RndMeth=Simplest
  Equal1 : RelationalOperator  Operator===  OutDataTypeStr=boolean  RndMeth=Simplest
  Equal2 : RelationalOperator  Operator===  OutDataTypeStr=boolean  RndMeth=Simplest
  Set Current Controller : Subsystem  TreatAsAtomicUnit=on
  Set Position Controller : Subsystem  TreatAsAtomicUnit=on
  Set Speed Controller : Subsystem  TreatAsAtomicUnit=on
  wires:
  Constant3/1 -> Equal1/2
  Equal2/1 -> Set Position Controller/Enable
  Equal/1 -> Set Current Controller/Enable
  Constant1/1 -> Equal2/2
  Constant/1 -> Equal/2
  Equal1/1 -> Set Speed Controller/Enable
  controllerSelection/1 -> Equal/1, Equal1/1, Equal2/1

== system Target_Control_System/Target_Control_System/InterruptFunction/pitchMotor_dataToMain/Variant Subsystem/Subsystem1 ==

== system Target_Control_System/Target_Control_System/InterruptFunction/pitchMotor_dataToMain/Variant Subsystem/VP_leader_follower_postion_copy ==
  Constant3 : Constant  Value=true
  Data Store Read24 : DataStoreRead  DataStoreName=oPitch  DataStoreElements=oPitch.oMot_.oParam_.uiSlaveRole_  IndexOptions=Index vector (dialog)  Indices=1  OutputSizes=1
  Follower Postion Enabled Subsystem : Subsystem  TreatAsAtomicUnit=on
  Leader Postion Enabled Subsystem : Subsystem  TreatAsAtomicUnit=on
  NOT1 : Logic  Operator=NOT  IconShape=distinctive  AllPortsSameDT=off  OutDataTypeStr=boolean
  Relational Operator : RelationalOperator  Operator===  OutDataTypeStr=boolean  RndMeth=Simplest
  wires:
  NOT1/1 -> Follower Postion Enabled Subsystem/Enable
  Relational Operator/1 -> Leader Postion Enabled Subsystem/Enable, NOT1/1
  Data Store Read24/1 -> Relational Operator/1
  Constant3/1 -> Relational Operator/2

== system Target_Control_System/Target_Control_System/InterruptFunction/pitchMotor_isrTask/abcToAlphaBeta/Alpha-Beta Calcs1 ==
  iInverseDirection : Inport
  fIa : Inport  Port=2
  fIb : Inport  Port=3
  fIc : Inport  Port=4
  fUaPostlpf : Inport  Port=5
  fUbPostlpf : Inport  Port=6
  fUcPostlpf : Inport  Port=7
  Demux1 : Demux  Outputs=2
  Demux4 : Demux  Outputs=2
  Mux1 : Mux  Inputs=3
  Mux3 : Mux  Inputs=3
  Switch : Switch  Criteria=u2 > Threshold
  Switch1 : Switch  Criteria=u2 > Threshold
  abc to alpha/beta1 : Gain  Gain="2/3*[1 -0.5 -0.5  ; 0 sqrt(3)/2 -sqrt(3)/2 ]"  Multiplication=Matrix(K*u) (u vector)
  abc to alpha/beta4 : Gain  Gain="2/3*[1 -0.5 -0.5  ; 0 sqrt(3)/2 -sqrt(3)/2 ]"  Multiplication=Matrix(K*u) (u vector)
  abc to alpha/beta_inverseDirection : Gain  Gain="2/3*[1 -0.5 -0.5  ; 0 -sqrt(3)/2 sqrt(3)/2 ]"  Multiplication=Matrix(K*u) (u vector)
  abc to alpha/beta_inverseDirection1 : Gain  Gain="2/3*[1 -0.5 -0.5  ; 0 -sqrt(3)/2 sqrt(3)/2 ]"  Multiplication=Matrix(K*u) (u vector)
  fIAlpha : Outport
  fIBeta : Outport  Port=2
  fUAlpha : Outport  Port=3
  fUBeta : Outport  Port=4
  wires:
  Demux4/1 -> fIAlpha/1
  Demux1/1 -> fUAlpha/1
  Demux1/2 -> fUBeta/1
  fIa/1 -> Mux1/1
  abc to alpha/beta1/1 -> Switch1/3
  abc to alpha/beta_inverseDirection1/1 -> Switch1/1
  Demux4/2 -> fIBeta/1
  Mux3/1 -> abc to alpha/beta_inverseDirection1/1, abc to alpha/beta1/1
  fUcPostlpf/1 -> Mux3/3
  fUbPostlpf/1 -> Mux3/2
  abc to alpha/beta_inverseDirection/1 -> Switch/1
  Switch1/1 -> Demux1/1
  abc to alpha/beta4/1 -> Switch/3
  fIc/1 -> Mux1/3
  Switch/1 -> Demux4/1
  iInverseDirection/1 -> Switch1/2, Switch/2
  Mux1/1 -> abc to alpha/beta4/1, abc to alpha/beta_inverseDirection/1
  fIb/1 -> Mux1/2
  fUaPostlpf/1 -> Mux3/1

== system Target_Control_System/Target_Control_System/InterruptFunction/pitchMotor_isrTask/abcToAlphaBeta/Calc Angle From Speed ==
  Omega : Inport
  Integrator with Angle Wrapper : Subsystem
  Integrator with Angle Wrapper_OLD : Subsystem  Commented=on
  fFluxMainAngleRaw2 : Outport
  wires:
  Omega/1 -> Integrator with Angle Wrapper/1(Omega)
  Integrator with Angle Wrapper/1(Angle) -> fFluxMainAngleRaw2/1  "fFluxMainAngleRaw2_"

== system Target_Control_System/Target_Control_System/InterruptFunction/pitchMotor_isrTask/abcToAlphaBeta/ModelSource ==
  note: 1) Add Subsystem or Model blocks as valid variant choices.
      | 2) You cannot connect blocks at this level. At simulation, connectivity is automatically
      | determined, based on the active variant and port name matching.
  DoNotIncludeCustomCode : Subsystem  TreatAsAtomicUnit=on  VariantControl=TARGET_CODE_GEN == 0
  IncludeCustomCode : Subsystem  TreatAsAtomicUnit=on  VariantControl=(default)

== system Target_Control_System/Target_Control_System/InterruptFunction/pitchMotor_isrTask/abcToAlphaBeta/vsincos()1 ==
  fUphFilterDelayAngleRad : Inport
  fFluxMainAngleRaw2 : Inport  Port=2
  Enable : EnablePort
  Cos : Trigonometry  Operator=cos
  Cos1 : Trigonometry  Operator=cos
  Data Store Write1 : DataStoreWrite  DataStoreName=mdl_pitch_fUphFilterDelayAngleRad_sin_  IndexOptions=Index vector (dialog)  Indices=1  OutputSizes=1
  Data Store Write2 : DataStoreWrite  DataStoreName=mdl_pitch_fUphFilterDelayAngleRad_cos_  IndexOptions=Index vector (dialog)  Indices=1  OutputSizes=1
  Data Store Write7 : DataStoreWrite  DataStoreName=mdl_pitch_fFluxMainAngleRaw2_sin_  IndexOptions=Index vector (dialog)  Indices=1  OutputSizes=1
  Data Store Write8 : DataStoreWrite  DataStoreName=mdl_pitch_fFluxMainAngleRaw2_cos_  IndexOptions=Index vector (dialog)  Indices=1  OutputSizes=1
  Sin : Trigonometry
  Sin1 : Trigonometry
  wires:
  fUphFilterDelayAngleRad/1 -> Sin/1, Cos/1
  fFluxMainAngleRaw2/1 -> Cos1/1, Sin1/1
  Cos/1 -> Data Store Write2/1
  Sin1/1 -> Data Store Write7/1
  Sin/1 -> Data Store Write1/1
  Cos1/1 -> Data Store Write8/1
